simulink library "INT_APP_DD2"  (R2016b)
settings: Solver=VariableStepAuto  StartTime=0.0  StopTime=10.0  RelTol=1e-3
settings Model: Creator=Administrator  LastModifiedBy=Administrator

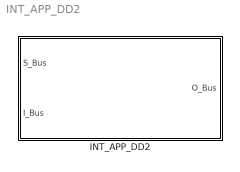
== system INT_APP_DD2 ==
  INT_APP_DD2 : Subsystem

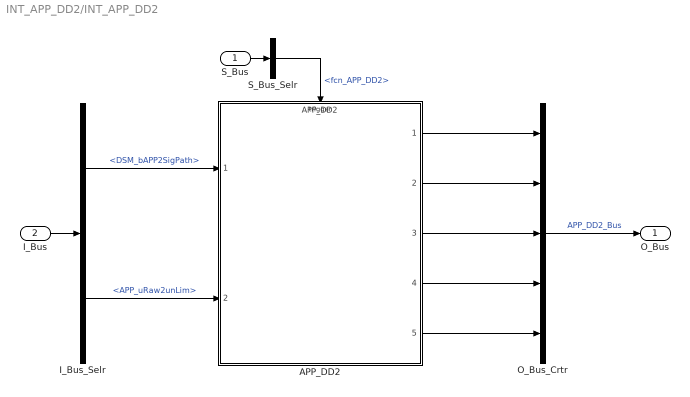
== system INT_APP_DD2/INT_APP_DD2 ==
  S_Bus : Inport
  I_Bus : Inport  Port=2
  APP_DD2 : ModelReference  ModelNameDialog=APP_DD2  SimulationMode=Normal  ModelReferenceVersion=1.14  TriggerPortName=function  TriggerPortTriggerType=function-call  TriggerPortStatesWhenEnabling=held
  I_Bus_Selr : BusSelector  OutputSignals=DSM_bAPP2SigPath,APP_uRaw2unLim
  O_Bus_Crtr : BusCreator  Inputs=5
  S_Bus_Selr : BusSelector  OutputSignals=fcn_APP_DD2
  O_Bus : Outport
  wires:
  S_Bus_Selr/1 -> APP_DD2/Trigger  "<fcn_APP_DD2>"
  S_Bus/1 -> S_Bus_Selr/1
  I_Bus/1 -> I_Bus_Selr/1
  I_Bus_Selr/1 -> APP_DD2/1  "<DSM_bAPP2SigPath>"
  I_Bus_Selr/2 -> APP_DD2/2  "<APP_uRaw2unLim>"
  O_Bus_Crtr/1 -> O_Bus/1  "APP_DD2_Bus"
  APP_DD2/1 -> O_Bus_Crtr/1
  APP_DD2/2 -> O_Bus_Crtr/2
  APP_DD2/3 -> O_Bus_Crtr/3
  APP_DD2/4 -> O_Bus_Crtr/4
  APP_DD2/5 -> O_Bus_Crtr/5
